simulink library "calculateTargetWaypointReelIn"  (R2018a)
settings: Solver=VariableStepAuto  StartTime=0.0  StopTime=10.0  RelTol=1e-3
settings Model: Creator=mitch  LastModifiedBy=M.Cobb

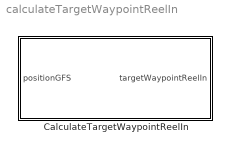
== system calculateTargetWaypointReelIn ==
  CalculateTargetWaypointReelIn : Subsystem

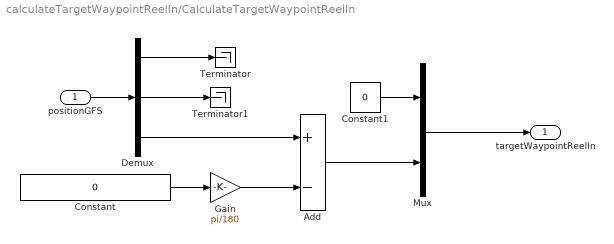
== system calculateTargetWaypointReelIn/CalculateTargetWaypointReelIn ==
  positionGFS : Inport
  Add : Sum  Inputs=+-
  Constant : Constant  Value=0
  Constant1 : Constant  Value=0
  Demux : Demux  Outputs=3
  Gain : Gain  Gain=pi/180
  Mux : Mux  Inputs=2
  Terminator : Terminator
  Terminator1 : Terminator
  targetWaypointReelIn : Outport
  wires:
  Gain/1 -> Add/2
  Constant/1 -> Gain/1
  Add/1 -> Mux/2
  Demux/3 -> Add/1
  Mux/1 -> targetWaypointReelIn/1
  Demux/1 -> Terminator/1
  positionGFS/1 -> Demux/1
  Demux/2 -> Terminator1/1
  Constant1/1 -> Mux/1
